simulink model "position_east_design"  (R2019b)
settings: Solver=FixedStepAuto  StartTime=0.0  StopTime=step_sim_time  FixedStep=1/step_sim_freq  RelTol=1e-3
values from neighbouring files (symbols this model uses):
  disturb = 1    [rootlocus.m]
  disturb_time = 20    [rootlocus.m]
  Kp_xe = 0.35    [rootlocus.m]
  step_time = 0    [rootlocus.m]
settings Model: Creator=francois  LastModifiedBy=francois

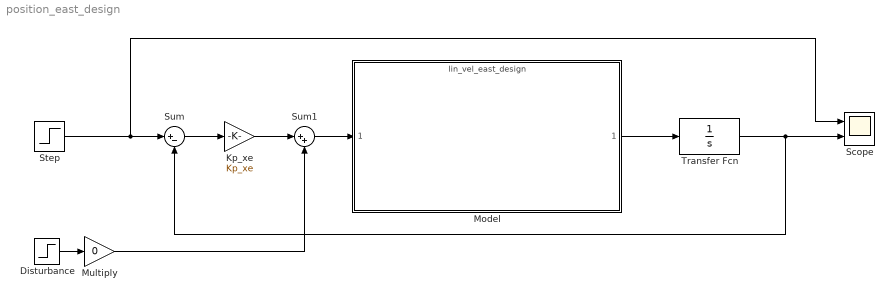
== system position_east_design ==
  "Disturbance " : Step  Time=disturb_time  After=disturb  SampleTime=0
  Kp_xe : Gain  Gain=Kp_xe
  Model : ModelReference  ModelNameDialog=lin_vel_east_design.slx  SimulationMode=Normal  ModelReferenceVersion=1.3
  Multiply : Gain  Gain=0
  Scope : Scope  NumInputPorts=2
  Step : Step  Time=step_time  SampleTime=0
  Sum : Sum  Inputs=|+-
  Sum1 : Sum  Inputs=|++
  Transfer Fcn : TransferFcn  Denominator=[1 0]
  wires:
  Sum1/1 -> Model/1
  Transfer Fcn/1 -> Sum/2, Scope/2
  Model/1 -> Transfer Fcn/1
  Sum/1 -> Kp_xe/1
  Kp_xe/1 -> Sum1/1
  Step/1 -> Scope/1, Sum/1
  "Disturbance "/1 -> Multiply/1
  Multiply/1 -> Sum1/2
